simulink model "Application_Problem_1_a"  (R2018b)
settings: Solver=VariableStepAuto  StartTime=0.0  StopTime=30  MaxStep=1e-3  RelTol=1e-3
StopFcn:
  | figure
  | set(groot,'defaultLineLineWidth',2)
  | set(groot,'defaultAxesFontWeight','bold')
  | 
  | subplot(4,1,1)
  | plot(Error_x,'LineWidth',2)
  | legend('x Error [m]')
  | grid on
  | subplot(4,1,2)
  | plot(Error_y,'LineWidth',2)
  | legend('y Error [m]')
  | grid on
  | subplot(4,1,3)
  | plot(PID_x,'LineWidth',2)
  | legend('PID x [degree]')
  | grid on
  | subplot(4,1,4)
  | plot(PID_y,'LineWidth',2)
  | legend('PID y [degree]')
  | grid on
  | xlabel('Time [sec]')
undefined symbols (not defined in the file or in its folder): X, Y, Z
libraries: nesl_utility x16, sm_lib x6, simulink x2
settings Model: Creator=nassi  LastModifiedBy=user
settings ExplorerConfigSet: InternalSimMechanicsExplorerSettings="<ExplorerConfiguration><canonicalview>default</canonicalview><AnimationSetting><BasePlaybackSpeed>1.0</BasePlaybackSpeed><PlaybackSpeedFactor>1.0</PlaybackSpeedFactor></AnimationSetting><TilePanel><TileInfo><Tiles Columns=\"2\" Count=\"4\" Rows=\"2\"><Column Weight=\"0.4993\"/><Column Weight=\"0.5007\"/><Row Weight=\"0.5\"/><Row Weight=\"0.5\"/><Tile Height=\"1\" Width=\"1\" X=\"0\" Y=\"0\"/><Tile Height=\"1\" Width=\"1\" X=\"0\" Y=\"1\"/><Tile Height=\"1\" Width=\"1\" X=\"1\" Y=\"0\"/><Tile Height=\"1\" Width=\"1\" X=\"1\" Y=\"1\"/></Tiles></TileInfo><SceneInfo><SceneViewer><BGColor><R>0.60000002384185791</R><G>0.60000002384185791</G><B>0.60000002384185791</B></BGColor><Camera><DoPerspective>off</DoPerspective><Position><X>0</X><Y>-1</Y><Z>0.0125940684229146616</Z></Position><Center><X>0</X><Y>-3.46944695195361419e-18</Y><Z>0.0125940684229146616</Z></Center><Up><X>0</X><Y>-0</Y><Z>1</Z></Up><ViewLimDist>1</ViewLimDist><YLim>0.177096935759567309</YLim><XLim>0.180249996930360784</XLim></Camera></SceneViewer><SceneViewer><BGColor><R>0.60000002384185791</R><G>0.60000002384185791</G><B>0.60000002384185791</B></BGColor><Camera><DoPerspective>off</DoPerspective><Position><X>0</X><Y>-1.73472347597680709e-18</Y><Z>1.01259408146143048</Z></Position><Center><X>0</X><Y>-1.73472347597680709e-18</Y><Z>0.0125940814614304841</Z></Center><Up><X>0</X><Y>1</Y><Z>-0</Z></Up><ViewLimDist>1</ViewLimDist><YLim>0.177096935759567309</YLim><XLim>0.180249996930360784</XLim></Camera></SceneViewer><SceneViewer><BGColor><R>0.60000002384185791</R><G>0.60000002384185791</G><B>0.60000002384185791</B></BGColor><Camera><DoPerspective>off</DoPerspective><Position><X>1</X><Y>0</Y><Z>0.0125940684229144395</Z></Position><Center><X>0</X><Y>0</Y><Z>0.0125940684229144395</Z></Center><Up><X>-0</X><Y>0</Y><Z>1</Z></Up><ViewLimDist>1</ViewLimDist><YLim>0.121084881014472179</YLim><XLim>0.123599997237324705</XLim></Camera></SceneViewer><SceneViewer><BGColor><R>0.60000002384185791</R><G>0.60000002384185791</G><B>0.60000002384185791</B></BGColor><Camera><DoPerspective>off</DoPerspective><Position><X>0.577350295265373403</X><Y>-0.577350295265373847</Y><Z>0.577350293503921197</Z></Position><Center><X>2.60757475331092228e-08</X><Y>-2.6075748004136959e-08</Y><Z>2.4314295350914229e-08</Z></Center><Up><X>-0.408248290463863073</X><Y>0.408248290463863073</Y><Z>0.816496580927726145</Z></Up><ViewLimDist>1</ViewLimDist><YLim>0.210482355646442548</YLim><XLim>0.21485439270734788</XLim></Camera></SceneViewer></SceneInfo></TilePanel><MechEditorPanel><Cameras/><GfxPanelCameraMap/><VideoCreator><PlaybackSpeedRatio>1.0</PlaybackSpeedRatio><FrameRate>30</FrameRate><VideoFormat>Motion JPEG AVI</VideoFormat><FrameSize>auto</FrameSize></VideoCreator></MechEditorPanel></ExplorerConfiguration>"

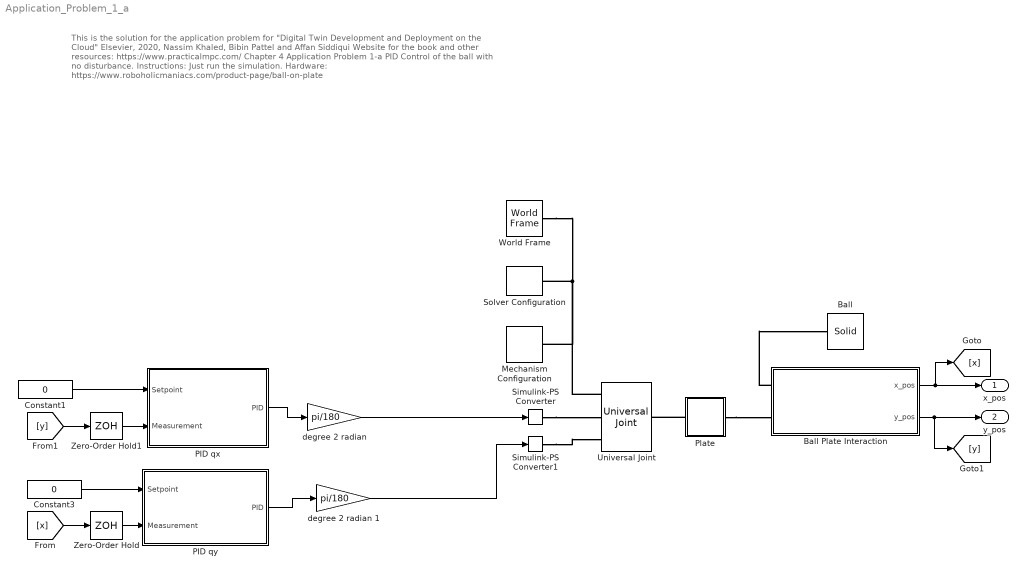
== system Application_Problem_1_a ==
  note: This is the solution for the application problem for "Digital Twin Development and Deployment on the Cloud" Elsevier, 2020, Nassim Khaled, Bibin Pattel and Affan Siddiqui
      |
      | Website for the book and other resources: https://www.practicalmpc.com/
      |
      | Chapter 4
      | Application Problem 1-a
      | PID Control of the ball with no disturbance.
      |
      | Instructions:
      | Just run the simulation.
      | Hardware: https://www.roboholicmaniacs.com/product-page/ball-on-plate
  Ball : sm_lib/Body Elements/Solid  InertiaType=CalculateFromGeometry  Mass=51  MassUnits=g  CenterOfMass=[0 0 0]  CenterOfMassUnits=m  MomentsOfInertia=[1 1 1]  MomentsOfInertiaUnits=kg*m^2  ProductsOfInertia=[0 0 0]  ProductsOfInertiaUnits=kg*m^2  BasedOnType=Mass  Density=1000  DensityUnits=kg/m^3  DoExposeReferenceFrame=on  SerializedFrames=<Frames/>  GraphicType=FromGeometry  MarkerShape=Sphere  MarkerSize=10  GraphicVisPropType=SimpleVisualProperties  GraphicDiffuseColor=[0.5 0.5 0.5]  GraphicSpecularColor=[0.5 0.5 0.5 1.0]  GraphicAmbientColor=[0.15 0.15 0.15 1.0]  GraphicEmissiveColor=[0.0 0.0 0.0 1.0]  GraphicShininess=75  GraphicOpacity=1.0  GeometryShape=Sphere  RectangleSize=[1 1]  RectangleSizeUnits=m  BrickDimensions=[1 1 1]  BrickDimensionUnits=m  CylinderRadius=1  CylinderRadiusUnits=m  CylinderLength=1  CylinderLengthUnits=m  SphereRadius=2.54/2  SphereRadiusUnits=cm  EllipsoidRadii=[1 1 1]  EllipsoidRadiiUnits=m  ExtrusionCrossSection=[1 1; -1 1; -1 -1; 1 -1]  ExtrusionCrossSectionUnits=m  ExtrusionLength=1  ExtrusionLengthUnits=m  PolygonNumSides=3  PolygonOuterRadius=1  PolygonOuterRadiusUnits=m  ExtGeomFileType=STEP  ExtGeomFileUnits=m  RevolutionCrossSection=[1 1; 1 -1; 2 -1; 2 1]  RevolutionCrossSectionUnits=m  RevolutionExtent=Full  RevolutionAngle=180  RevolutionAngleUnits=deg
  Ball Plate Interaction : Subsystem
  Constant1 : Constant  Value=0
  Constant3 : Constant  Value=0
  Mechanism Configuration : sm_lib/Utilities/Mechanism Configuration  UniformGravity=Constant  GravityVector=[0 0 -9.81]  GravityUnits=m/s^2  LinearizationDelta=0.001
  PID qx : Subsystem
  PID qy : Subsystem
  Plate : Subsystem
  Simulink-PS Converter : nesl_utility/Simulink-PS Converter  PhysicalDomain=network_engine_domain  SubClassName=ps_input  LeftPortType=input  RightPortType=output  PseudoPeriodic=off  Frequencies=[]  NoiseDistribution=none  NoiseParameters=[]  Unit=1  AffineConversion=off  FilteringAndDerivatives=zero  SimscapeFilterOrder=1  InputFilterTimeConstant=0.001  UdotUserProvided=0
  Simulink-PS Converter1 : nesl_utility/Simulink-PS Converter  PhysicalDomain=network_engine_domain  SubClassName=ps_input  LeftPortType=input  RightPortType=output  PseudoPeriodic=off  Frequencies=[]  NoiseDistribution=none  NoiseParameters=[]  Unit=1  AffineConversion=off  FilteringAndDerivatives=zero  SimscapeFilterOrder=1  InputFilterTimeConstant=0.001  UdotUserProvided=0
  Solver Configuration : nesl_utility/Solver Configuration  PhysicalDomain=network_engine_domain  SubClassName=solver  LeftPortType=input  RightPortType=generic  Tones=[]  Harmonics=[]  SimulateNoise=off  Profile=off  UseLocalSampling=off  EnableSwitchedLinearOptims=on  FrequencyDomain=off  UseCCode=off  RelTol=0.001  AbsTol=1e-06  MinStep=1e-09  ToWorkspace=off  RevertToSquareIcSolve=off  NumHomotopyIterations=100  PhasorMode=off  PhasorModeNumHarmonics=1  DoDC=off  ResidualTolerance=1e-9  UseLocalSolver=off  LocalSolverChoice=NE_BACKWARD_EULER_ADVANCER  LocalSolverSampleTime=.001  DoFixedCost=off  MaxNonlinIter=3  MaxModeIter=2  LinearAlgebra=Sparse  EquationFormulation=NE_TIME_EF  DelaysMemoryBudget=1024  AutomaticFiltering=on  FilteringTimeConstant=0.001  PartitionStorageMethod=AS_NEEDED  PartitionMemoryBudget=1024
  Universal Joint : sm_lib/Joints/Universal Joint  SenseConstraintForce=off  SenseConstraintForceX=off  SenseConstraintForceY=off  SenseConstraintForceZ=off  SenseConstraintTorque=off  SenseConstraintTorqueX=off  SenseConstraintTorqueY=off  SenseConstraintTorqueZ=off  SenseTotalForce=off  SenseTotalForceX=off  SenseTotalForceY=off  SenseTotalForceZ=off  SenseTotalTorque=off  SenseTotalTorqueX=off  SenseTotalTorqueY=off  SenseTotalTorqueZ=off  CompositeWrenchDir=FollowerOnBase  CompositeWrenchFrame=BaseFrame  RxEquilibriumPosition=0  RxEquilibriumPositionUnits=deg  RxSpringStiffness=0  RxSpringStiffnessUnits=N*m/deg  RxDampingCoefficient=0  RxDampingCoefficientUnits=N*m/(deg/s)  RxTorqueActuationMode=ComputedTorque  RxMotionActuationMode=InputMotion  RxSensePosition=off  RxSenseVelocity=off  RxSenseAcceleration=off  RxSenseTorqueForce=off  RxPositionTargetSpecify=off  RxPositionTargetPriority=High  RxPositionTargetValue=0  RxPositionTargetValueUnits=deg  RxVelocityTargetSpecify=off  RxVelocityTargetPriority=High  RxVelocityTargetValue=0  RxVelocityTargetValueUnits=deg/s  RyEquilibriumPosition=0  RyEquilibriumPositionUnits=deg  RySpringStiffness=0  RySpringStiffnessUnits=N*m/deg  RyDampingCoefficient=0  RyDampingCoefficientUnits=N*m/(deg/s)  RyTorqueActuationMode=ComputedTorque  RyMotionActuationMode=InputMotion  RySensePosition=off  RySenseVelocity=off  RySenseAcceleration=off  RySenseTorqueForce=off  RyPositionTargetSpecify=off  RyPositionTargetPriority=High  RyPositionTargetValue=0  RyPositionTargetValueUnits=deg  RyVelocityTargetSpecify=off  RyVelocityTargetPriority=High  RyVelocityTargetValue=0  RyVelocityTargetValueUnits=deg/s
      settings: SourceProductName=Simscape Multibody
  World Frame : sm_lib/Frames and Transforms/World Frame
  Zero-Order Hold : ZeroOrderHold  SampleTime=0.1
  Zero-Order Hold1 : ZeroOrderHold  SampleTime=0.1
  degree 2 radian : Gain  Gain=pi/180
  degree 2 radian 1 : Gain  Gain=pi/180
  x_pos : Outport
  y_pos : Outport  Port=2
  wires:
  Ball Plate Interaction/1(x_pos) -> [x], x_pos/1
  Ball Plate Interaction/2(y_pos) -> [y], y_pos/1
  [x] -> Zero-Order Hold/1
  [y] -> Zero-Order Hold1/1
  degree 2 radian/1 -> Simulink-PS Converter/1
  degree 2 radian 1/1 -> Simulink-PS Converter1/1
  PID qx/1(PID) -> degree 2 radian/1
  PID qy/1(PID) -> degree 2 radian 1/1
  Zero-Order Hold/1 -> PID qy/2(Measurement)
  Constant3/1 -> PID qy/1(Setpoint)
  Zero-Order Hold1/1 -> PID qx/2(Measurement)
  Constant1/1 -> PID qx/1(Setpoint)
  connections:
  World Frame/RConn1 -- Mechanism Configuration/RConn1 -- Universal Joint/LConn1 -- Solver Configuration/RConn1
  Plate/LConn1 -- Universal Joint/RConn1
  Ball Plate Interaction/LConn1 -- Ball/RConn1
  Plate/RConn1 -- Ball Plate Interaction/LConn2
  Simulink-PS Converter/RConn1 -- Universal Joint/LConn2
  Simulink-PS Converter1/RConn1 -- Universal Joint/LConn3

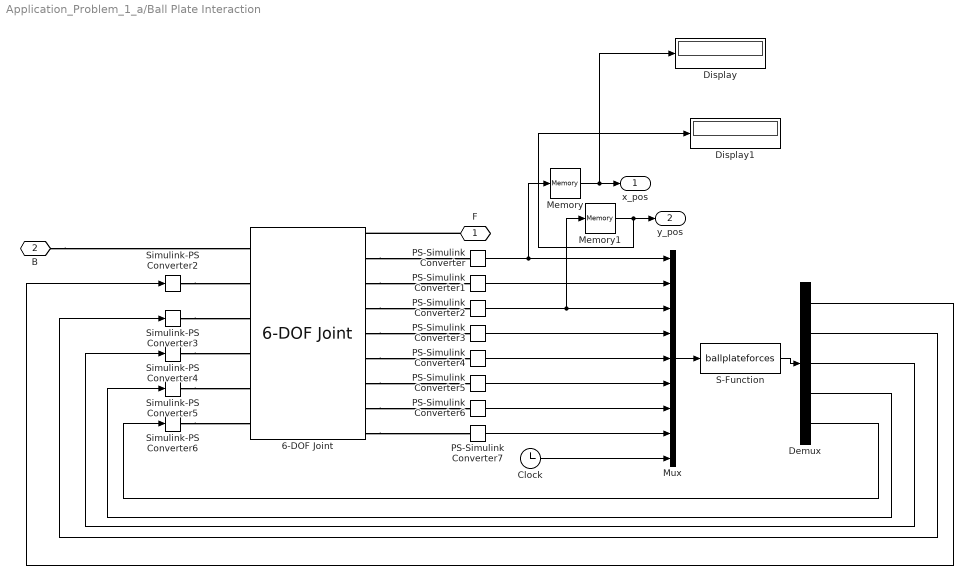
== system Application_Problem_1_a/Ball Plate Interaction ==
  6-DOF Joint : sm_lib/Joints/6-DOF Joint  SenseConstraintForce=off  SenseConstraintForceX=off  SenseConstraintForceY=off  SenseConstraintForceZ=off  SenseConstraintTorque=off  SenseConstraintTorqueX=off  SenseConstraintTorqueY=off  SenseConstraintTorqueZ=off  SenseTotalForce=off  SenseTotalForceX=off  SenseTotalForceY=off  SenseTotalForceZ=off  SenseTotalTorque=off  SenseTotalTorqueX=off  SenseTotalTorqueY=off  SenseTotalTorqueZ=off  CompositeWrenchDir=FollowerOnBase  CompositeWrenchFrame=BaseFrame  PxEquilibriumPosition=0  PxEquilibriumPositionUnits=m  PxSpringStiffness=0  PxSpringStiffnessUnits=N/m  PxDampingCoefficient=0  PxDampingCoefficientUnits=N/(m/s)  PxTorqueActuationMode=InputTorque  PxMotionActuationMode=ComputedMotion  PxSensePosition=on  PxSenseVelocity=on  PxSenseAcceleration=off  PxSenseTorqueForce=off  PxPositionTargetSpecify=off  PxPositionTargetPriority=High  PxPositionTargetValue=0  PxPositionTargetValueUnits=m  PxVelocityTargetSpecify=off  PxVelocityTargetPriority=High  PxVelocityTargetValue=0  PxVelocityTargetValueUnits=m/s  PyEquilibriumPosition=0  PyEquilibriumPositionUnits=m  PySpringStiffness=0  PySpringStiffnessUnits=N/m  PyDampingCoefficient=0  PyDampingCoefficientUnits=N/(m/s)  PyTorqueActuationMode=InputTorque  PyMotionActuationMode=ComputedMotion  PySensePosition=on  PySenseVelocity=on  PySenseAcceleration=off  PySenseTorqueForce=off  PyPositionTargetSpecify=off  PyPositionTargetPriority=High  PyPositionTargetValue=0  PyPositionTargetValueUnits=m  PyVelocityTargetSpecify=off  PyVelocityTargetPriority=High  PyVelocityTargetValue=0  PyVelocityTargetValueUnits=m/s  PzEquilibriumPosition=0  PzEquilibriumPositionUnits=m  PzSpringStiffness=0  PzSpringStiffnessUnits=N/m  PzDampingCoefficient=0  PzDampingCoefficientUnits=N/(m/s)  PzTorqueActuationMode=InputTorque  PzMotionActuationMode=ComputedMotion  PzSensePosition=on  PzSenseVelocity=on  PzSenseAcceleration=off  PzSenseTorqueForce=off  PzPositionTargetSpecify=on  PzPositionTargetPriority=High  PzPositionTargetValue=0.0227  PzPositionTargetValueUnits=m  PzVelocityTargetSpecify=off  PzVelocityTargetPriority=High  PzVelocityTargetValue=0  PzVelocityTargetValueUnits=m/s  SphDefPosRotationMethod=None  SphDefPosRotationAngleUnits=deg  SphDefPosRotationStandardAxis=+Z  SphDefPosRotationAngle=0.0  SphDefPosRotationArbitraryAxis=[0 0 1]  SphDefPosFollAlignAxisA=+X  SphDefPosBaseAlignAxisA=+Y  SphDefPosFollAlignAxisB=+Y  SphDefPosBaseAlignAxisB=+Z  SphDefPosRotationSequenceAxes=FollowerAxes  SphDefPosRotationSequence=XYX  SphDefPosRotationSequenceAngles=[0 0 0]  SphDefPosRotationSequenceAnglesUnits=deg  SphDefPosRotationMatrix=[1 0 0; 0 1 0; 0 0 1]  SphEqPosRotationMethod=None  SphEqPosRotationAngleUnits=deg  SphEqPosRotationStandardAxis=+Z  SphEqPosRotationAngle=0.0  SphEqPosRotationArbitraryAxis=[0 0 1]  SphEqPosFollAlignAxisA=+X  SphEqPosBaseAlignAxisA=+Y  SphEqPosFollAlignAxisB=+Y  SphEqPosBaseAlignAxisB=+Z  SphEqPosRotationSequenceAxes=FollowerAxes  SphEqPosRotationSequence=XYX  SphEqPosRotationSequenceAngles=[0 0 0]  SphEqPosRotationSequenceAnglesUnits=deg  SphEqPosRotationMatrix=[1 0 0; 0 1 0; 0 0 1]  SphSpringStiffness=0  SphSpringStiffnessUnits=N*m/deg  SphDampingCoefficient=0  SphDampingCoefficientUnits=N*m/(deg/s)  SphActuateTorqueX=on  SphActuateTorqueY=on  SphActuateTorqueZ=off  SphActuateTorque=off  SphTorqueActuationMode=InputTorque  SphMotionActuationMode=ComputedMotion  SphActuationFrame=BaseFrame  SphSensePosition=off  SphSenseVelocityX=on  SphSenseVelocityY=on  SphSenseVelocityZ=off  SphSenseVelocity=off  SphSenseAccelerationX=off  SphSenseAccelerationY=off  SphSenseAccelerationZ=off  SphSenseAcceleration=off  SphSenseTorqueX=off  SphSenseTorqueY=off  SphSenseTorqueZ=off  SphSenseTorqueForce=off  SphSensingFrame=BaseFrame  SphPositionTargetRotationMethod=None  SphPositionTargetRotationAngleUnits=deg  SphPositionTargetRotationStandardAxis=+Z  SphPositionTargetRotationAngle=0.0  SphPositionTargetRotationArbitraryAxis=[0 0 1]  SphPositionTargetFollAlignAxisA=+X  SphPositionTargetBaseAlignAxisA=+Y  SphPositionTargetFollAlignAxisB=+Y  SphPositionTargetBaseAlignAxisB=+Z  SphPositionTargetRotationSequenceAxes=FollowerAxes  SphPositionTargetRotationSequence=XYX  SphPositionTargetRotationSequenceAngles=[0 0 0]  SphPositionTargetRotationSequenceAnglesUnits=deg  SphPositionTargetRotationMatrix=[1 0 0; 0 1 0; 0 0 1]  SphPositionTargetSpecify=off  SphPositionTargetPriority=High  SphVelocityTargetValue=[0 0 0]  SphVelocityTargetValueUnits=deg/s  SphVelocityTargetSpecify=off  SphVelocityTargetPriority=High  SphVelocityTargetInFollowerFrame=on
  Clock : Clock
  Demux : Demux  Outputs=5
  Display : Display
  Display1 : Display
  Memory : Memory
  Memory1 : Memory
  Mux : Mux  Inputs=9
  PS-Simulink Converter{,1..7} (8 alike) : nesl_utility/PS-Simulink Converter  PhysicalDomain=network_engine_domain  SubClassName=ps_output  LeftPortType=input  RightPortType=output  PseudoPeriodic=off  Frequencies=[]  Unit=1  AffineConversion=off
  S-Function : S-Function  FunctionName=ballplateforces  Parameters=0.35,0.24, 0.02, 0.0254/2, 1000, 100, 0.6, 1e-4  SFunctionDeploymentMode=off  EnableBusSupport=off
  Simulink-PS Converter{2..6} (5 alike) : nesl_utility/Simulink-PS Converter  PhysicalDomain=network_engine_domain  SubClassName=ps_input  LeftPortType=input  RightPortType=output  PseudoPeriodic=off  Frequencies=[]  NoiseDistribution=none  NoiseParameters=[]  Unit=1  AffineConversion=off  FilteringAndDerivatives=provide  SimscapeFilterOrder=1  InputFilterTimeConstant=0.001  UdotUserProvided=0
  F : PMIOPort  Side=Left
  B : PMIOPort  Port=2  Side=Left
  x_pos : Outport
  y_pos : Outport  Port=2
  wires:
  PS-Simulink Converter2/1 -> Memory1/1, Mux/3
  Demux/4 -> Simulink-PS Converter5/1
  PS-Simulink Converter7/1 -> Mux/8
  PS-Simulink Converter3/1 -> Mux/4
  Demux/5 -> Simulink-PS Converter6/1
  S-Function/1 -> Demux/1
  PS-Simulink Converter5/1 -> Mux/6
  PS-Simulink Converter/1 -> Memory/1, Mux/1
  PS-Simulink Converter1/1 -> Mux/2
  Clock/1 -> Mux/9
  PS-Simulink Converter6/1 -> Mux/7
  PS-Simulink Converter4/1 -> Mux/5
  Demux/3 -> Simulink-PS Converter4/1
  Demux/2 -> Simulink-PS Converter3/1
  Mux/1 -> S-Function/1
  Memory/1 -> Display/1, x_pos/1
  Memory1/1 -> Display1/1, y_pos/1
  Demux/1 -> Simulink-PS Converter2/1
  connections:
  6-DOF Joint/RConn7 -- PS-Simulink Converter5/LConn1
  Simulink-PS Converter5/RConn1 -- 6-DOF Joint/LConn5
  F/RConn1 -- 6-DOF Joint/RConn1
  B/RConn1 -- 6-DOF Joint/LConn1
  Simulink-PS Converter6/RConn1 -- 6-DOF Joint/LConn6
  6-DOF Joint/RConn6 -- PS-Simulink Converter4/LConn1
  Simulink-PS Converter3/RConn1 -- 6-DOF Joint/LConn3
  6-DOF Joint/RConn3 -- PS-Simulink Converter1/LConn1
  6-DOF Joint/RConn5 -- PS-Simulink Converter3/LConn1
  Simulink-PS Converter4/RConn1 -- 6-DOF Joint/LConn4
  6-DOF Joint/RConn4 -- PS-Simulink Converter2/LConn1
  Simulink-PS Converter2/RConn1 -- 6-DOF Joint/LConn2
  6-DOF Joint/RConn9 -- PS-Simulink Converter7/LConn1
  6-DOF Joint/RConn8 -- PS-Simulink Converter6/LConn1
  6-DOF Joint/RConn2 -- PS-Simulink Converter/LConn1

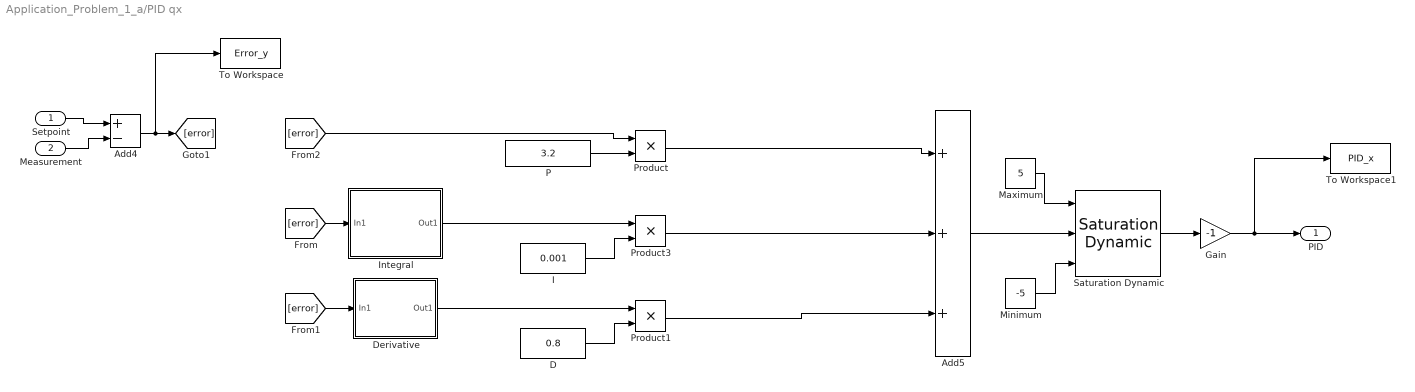
== system Application_Problem_1_a/PID qx ==
  Setpoint : Inport
  Measurement : Inport  Port=2
  Add4 : Sum  Inputs=+-
  Add5 : Sum  Inputs=+++
  D : Constant  Value=0.8
  Derivative : Subsystem
  Gain : Gain  Gain=-1
  I : Constant  Value=0.001
  Integral : Subsystem
  Maximum : Constant  Value=5
  Minimum : Constant  Value=-5
  P : Constant  Value=3.2
  Product : Product
  Product1 : Product
  Product3 : Product
  Saturation Dynamic : simulink/Discontinuities/Saturation Dynamic  OutMin=[]  OutMax=[]  OutDataTypeStr=Inherit: Same as second input  OutDataType=fixdt(1, 16)  OutScaling=2^-10  DoSatur=off
  To Workspace : ToWorkspace  VariableName=Error_y  SaveFormat=Timeseries  SampleTime=0.1
  To Workspace1 : ToWorkspace  VariableName=PID_x  SaveFormat=Timeseries  SampleTime=0.1
  PID : Outport
  wires:
  P/1 -> Product/2
  Minimum/1 -> Saturation Dynamic/3
  Maximum/1 -> Saturation Dynamic/1
  D/1 -> Product1/2
  I/1 -> Product3/2
  Add4/1 -> To Workspace/1, [error]
  Product/1 -> Add5/1
  Product3/1 -> Add5/2
  Product1/1 -> Add5/3
  Saturation Dynamic/1 -> Gain/1
  Setpoint/1 -> Add4/1
  Measurement/1 -> Add4/2
  [error] -> Integral/1(In1)
  Integral/1(Out1) -> Product3/1
  [error] -> Product/1
  [error] -> Derivative/1(In1)
  Derivative/1(Out1) -> Product1/1
  Add5/1 -> Saturation Dynamic/2
  Gain/1 -> To Workspace1/1, PID/1

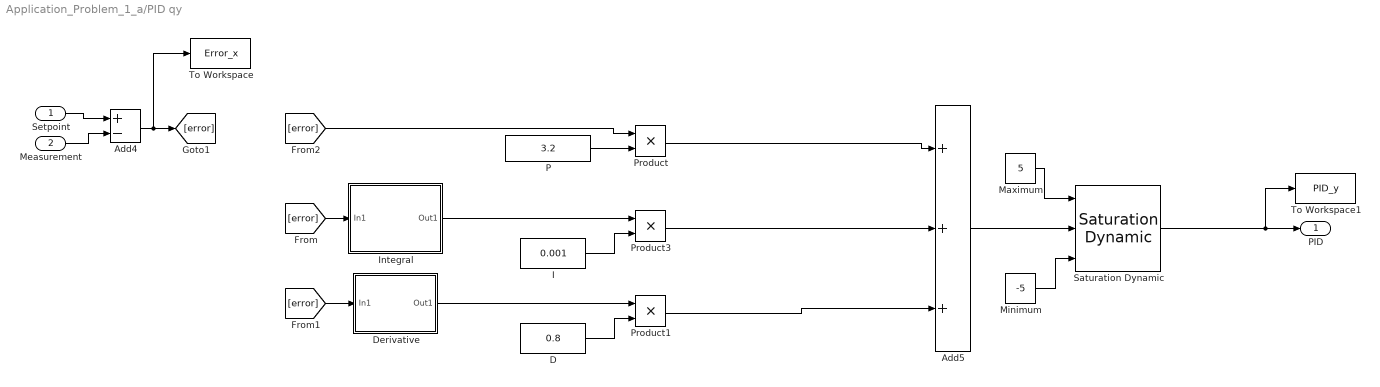
== system Application_Problem_1_a/PID qy ==
  Setpoint : Inport
  Measurement : Inport  Port=2
  Add4 : Sum  Inputs=+-
  Add5 : Sum  Inputs=+++
  D : Constant  Value=0.8
  Derivative : Subsystem
  I : Constant  Value=0.001
  Integral : Subsystem
  Maximum : Constant  Value=5
  Minimum : Constant  Value=-5
  P : Constant  Value=3.2
  Product : Product
  Product1 : Product
  Product3 : Product
  Saturation Dynamic : simulink/Discontinuities/Saturation Dynamic  OutMin=[]  OutMax=[]  OutDataTypeStr=Inherit: Same as second input  OutDataType=fixdt(1, 16)  OutScaling=2^-10  DoSatur=off
  To Workspace : ToWorkspace  VariableName=Error_x  SaveFormat=Timeseries  SampleTime=0.1
  To Workspace1 : ToWorkspace  VariableName=PID_y  SaveFormat=Timeseries  SampleTime=0.1
  PID : Outport
  wires:
  Add5/1 -> Saturation Dynamic/2
  Derivative/1(Out1) -> Product1/1
  [error] -> Derivative/1(In1)
  [error] -> Product/1
  Integral/1(Out1) -> Product3/1
  [error] -> Integral/1(In1)
  Measurement/1 -> Add4/2
  Setpoint/1 -> Add4/1
  Saturation Dynamic/1 -> To Workspace1/1, PID/1
  Product1/1 -> Add5/3
  Product3/1 -> Add5/2
  Product/1 -> Add5/1
  Add4/1 -> To Workspace/1, [error]
  I/1 -> Product3/2
  D/1 -> Product1/2
  Maximum/1 -> Saturation Dynamic/1
  Minimum/1 -> Saturation Dynamic/3
  P/1 -> Product/2

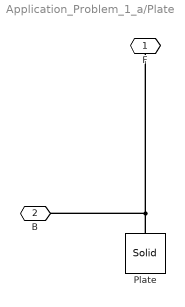
== system Application_Problem_1_a/Plate ==
  Plate : sm_lib/Body Elements/Solid  InertiaType=CalculateFromGeometry  Mass=1  MassUnits=kg  CenterOfMass=[0 0 0]  CenterOfMassUnits=m  MomentsOfInertia=[1 1 1]  MomentsOfInertiaUnits=kg*m^2  ProductsOfInertia=[0 0 0]  ProductsOfInertiaUnits=kg*m^2  BasedOnType=Density  Density=1.18  DensityUnits=g/cm^3  DoExposeReferenceFrame=on  SerializedFrames=<Frames/>  GraphicType=FromGeometry  MarkerShape=Sphere  MarkerSize=10  MarkerSizeUnits=m  GraphicVisPropType=SimpleVisualProperties  GraphicDiffuseColor=[0.5 0.5 0.5]  GraphicSpecularColor=[0.5 0.5 0.5 1.0]  GraphicAmbientColor=[0.15 0.15 0.15 1.0]  GraphicEmissiveColor=[0.0 0.0 0.0 1.0]  GraphicShininess=75  GraphicOpacity=1  GeometryShape=Brick  RectangleSize=[1 1]  RectangleSizeUnits=m  BrickDimensions=[0.35 0.24 0.02]  BrickDimensionUnits=m  CylinderRadius=1  CylinderRadiusUnits=m  CylinderLength=1  CylinderLengthUnits=m  SphereRadius=1  SphereRadiusUnits=m  EllipsoidRadii=[1 1 1]  EllipsoidRadiiUnits=m  ExtrusionCrossSection=[1 1; -1 1; -1 -1; 1 -1]  ExtrusionCrossSectionUnits=m  ExtrusionLength=1  ExtrusionLengthUnits=m  PolygonNumSides=3  PolygonOuterRadius=1  PolygonOuterRadiusUnits=m  ExtGeomFileType=STL  ExtGeomFileUnits=m  RevolutionCrossSection=[1 1; 1 -1; 2 -1; 2 1]  RevolutionCrossSectionUnits=m  RevolutionExtent=Full  RevolutionAngle=180  RevolutionAngleUnits=deg
  F : PMIOPort  Side=Right
  B : PMIOPort  Port=2  Side=Left
  connections:
  Plate/RConn1 -- F/RConn1 -- B/RConn1

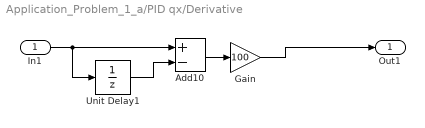
== system Application_Problem_1_a/PID qx/Derivative ==
  In1 : Inport
  Add10 : Sum  Inputs=+-
  Gain : Gain  Gain=100
  Unit Delay1 : UnitDelay  SampleTime=-1
  Out1 : Outport
  wires:
  Add10/1 -> Gain/1
  In1/1 -> Unit Delay1/1, Add10/1
  Unit Delay1/1 -> Add10/2
  Gain/1 -> Out1/1

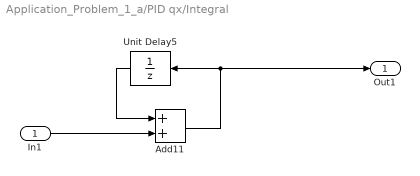
== system Application_Problem_1_a/PID qx/Integral ==
  In1 : Inport
  Add11 : Sum
  Unit Delay5 : UnitDelay  SampleTime=-1
  Out1 : Outport
  wires:
  Unit Delay5/1 -> Add11/1
  Add11/1 -> Out1/1, Unit Delay5/1
  In1/1 -> Add11/2

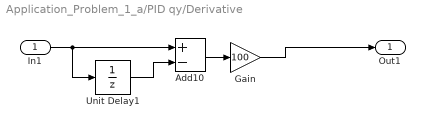
== system Application_Problem_1_a/PID qy/Derivative ==
  In1 : Inport
  Add10 : Sum  Inputs=+-
  Gain : Gain  Gain=100
  Unit Delay1 : UnitDelay  SampleTime=-1
  Out1 : Outport
  wires:
  Gain/1 -> Out1/1
  Unit Delay1/1 -> Add10/2
  In1/1 -> Add10/1, Unit Delay1/1
  Add10/1 -> Gain/1

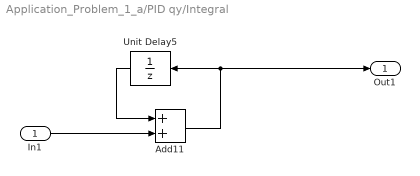
== system Application_Problem_1_a/PID qy/Integral ==
  In1 : Inport
  Add11 : Sum
  Unit Delay5 : UnitDelay  SampleTime=-1
  Out1 : Outport
  wires:
  In1/1 -> Add11/2
  Add11/1 -> Unit Delay5/1, Out1/1
  Unit Delay5/1 -> Add11/1
